simulink model "Predefined_with_GroundTruth_mod1helper"  (R2021b)
settings: Solver=VariableStepAuto  StartTime=0.0  StopTime=inf  RelTol=1e-3
model workspace (MAT data in the model file):
  firstWarning = 1
  originalScenarioChecksum = '114339432DE22364D47BB28FC96DC10C'
undefined symbols (not defined in the file): Acceleration, ActorID, AngularVelocity, curvature, curvature1, curvatureAhd, DefaultGear, DEND_B, DEND_S, DEND_T, direction, driving, EgoRefPose, gradbp, L, LF, LR, matlabshared, MAX_BRAKE, MAX_STEER, MAX_TORQUE, MCAR, MIN_BRAKE, MIN_STEER, MIN_TORQUE, NUMD_B, NUMD_S, NUMD_T, Pitch, Position, psi_o, R, Roll, RRdamp, scenario, SceneInfo, sigbuilder_block, STEER_RATIO, stopSign_ID, Tdead, thetaRefs, TL_ID, TrackWidth, Ts, ts, Vdead, Velocity, VelProfile, X_o, xRef2s, Y_o, Yaw, yRef2s
libraries: drivingscenarioandsensors x8, drivingvehiclecontroller x2, simulink x2, trackingutilitieslib x2, mpcadaslib x1, robotalgslib x1, simulink_extras x1, drivinglib x1, autolibshared x1, vehdynlibviscommon x1, vehdynlibsteering x1
(part 1 of 3)
settings Model: Creator=akshran  LastModifiedBy=almudhaf.3

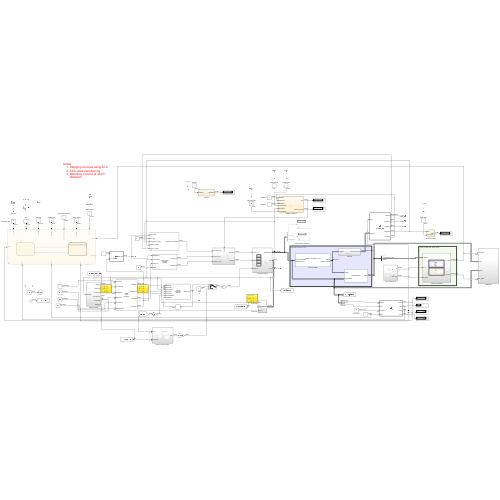
[thumbnail: Simulink's stored preview of the top-level diagram]
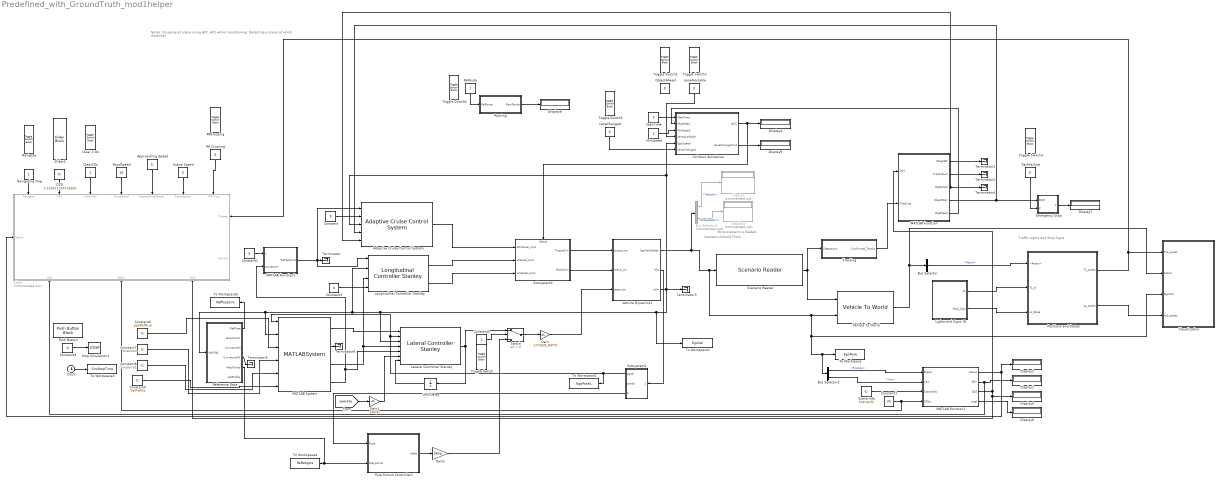
== system Predefined_with_GroundTruth_mod1helper ==
  note: Notes:
      | Stopping at scene using ACC.
      | ACC while transitioning.
      | Detecting a scene at which distance?
  note: Mcity scenario is loaded
  note: Traffic Lights and Stop Signs
  note: Scenario Ground Truth
  Adaptive Cruise Control System : mpcadaslib/Adaptive Cruise Control System  EgoModel=tf(1,[0.5,1,0])  InitialEgoVelocity=0  DefaultSpacing=2  MaxVelocity=50  MinAcceleration=-6  amin_ext=off  MaxAcceleration=6  amax_ext=off  Ts=0.1  PredictionHorizon=30  ControllerBehavior=0.500  suboptimal=off  maxiter=10  datatypeopt=double  optmode=off  trackmode=off
  Approaching Speed : Constant  Value=5
  Bus Selector : BusSelector  OutputSignals=Actors
  Bus Selector2 : BusSelector  OutputSignals=Position,Yaw
  Bus Selector4 : BusSelector  Commented=on  OutputSignals=Velocity,Acceleration
  Chart : Stateflow chart  Commented=on  TreatAsAtomicUnit=on
      settings: PortSchema="{\"entries\":[{\"content\":{\"sides\":[{\"content\":{\"connectorIds\":[\"In8\"]},\"type\":\"ConnectorPlacement.EquallySpacedRectSide\",\"uuid\":\"81aca70f-0947-49fb-b60a-be241e44193b\"},{\"content\":{\"connectorIds\":[\"In1\",\"Out1\"],\"side\":\"RIGHT\"},\"type\":\"ConnectorPlacement.EquallySpacedRectSide\",\"uuid\":\"e7b9645e-3711-4964-ac9b-0199dd335e99\"},{\"content\":{\"connectorIds\":[\"In9\",\"In10\",\"In11\",\"In12\",\"In3\",\"In4\",\"In6\"],\"side\":\"TOP\"},\"type\":\"ConnectorPlacement.EquallySpacedRectSide\",\"uuid\":\"6876f024-944b-4540-9404-d68f37763657\"},{\"content\":{\"connectorIds\":[\"In2\",\"In5\",\"In7\"],\"side\":\"BOTTOM\"},\"type\":\"ConnectorPlacement.EquallySpacedRectSide\",\"uuid\":\"44acab73-cdde-4edf-95df-27422644ccab\"}]},\"type\":\"ConnectorPlacement.EquallySpacedConnector\",\"uuid\":\"d2c31c01-e447-43db-8d2b-8b98a0ca291a\"}],\"packageUris\":[\"http://schema.mathworks.com/mf0/Connector/R2020b\"],\"version\":\"1.0\"}"
  Clear 2 Go : ToggleSwitchBlock
      settings: Values={{'Off', 'On'}, [0 1]}
  Clear2Go : Constant
  Clock : Clock
  Collision Avoidance : Stateflow chart  TreatAsAtomicUnit=on
  Constant : Constant  Value=0
  Constant1 : Constant  Value=25
  Constant2 : Constant  Value=5
  Constant3 : Constant  Value=0
  Constant4 : Constant  Value=0
  Constant5 : Constant
  Constant6 : Constant  Value=EgoRefPose
  Constant7 : Constant  Value=direction
  Constant8 : Constant  Value=curvature1
  Constant9 : Constant  Value=VelProfile
  D2D : Constant  Value=2.529411764705882
  Display : Display  Commented=on
  Display{1..2,4..9} (8 alike) : Display
  Display3 : Display  Commented=on
  Emergency Stop : Stateflow chart  TreatAsAtomicUnit=on
  Gain : Gain  Gain=1/STEER_RATIO
  Gain1 : Gain  Gain=180/pi
  Gain2 : Gain  Gain=180/pi
  LaneAvailable : Constant  Value=0
  LaneChanged : Constant  Value=0
  Lateral Controller Stanley : drivingvehiclecontroller/Lateral Controller Stanley  ModelType=Dynamic bicycle model  PositionGainF=2.5  PositionGainR=2.5  YawRateGain=0.4  DelayGain=0.4  VehicleMass=MCAR  Lf=LF  Lr=LR  TireStiffness=5e3  Wheelbase=3  MaxSteeringAngle=80
      settings: SourceProductBaseCode=DR
  Lights and Signs ID : Subsystem
  Longitudinal Controller Stanley : drivingvehiclecontroller/Longitudinal Controller Stanley  Kp=10  Ki=0.1  SampleTime=0.05  MaxAcceleration=40  MaxDeceleration=40
      settings: SourceProductBaseCode=DR
  MATLAB Function : MATLAB Function  TreatAsAtomicUnit=on
  MATLAB Function1 : MATLAB Function  TreatAsAtomicUnit=on
  MATLAB Function2 : MATLAB Function  TreatAsAtomicUnit=on
  MATLAB System : MATLABSystem  System=HelperPathAnalyzer  Wheelbase=WB  HasResetOutput=off  SimulateUsing=Interpreted execution
      mask Type: HelperPathAnalyzer
      mask Display:
      | disp(['Helper' char(10) 'Path' char(10) 'Analyzer']);
      | port_label('input',1,'CurrPose');
      | port_label('input',2,'CurrVelocity');
      | port_label('input',3,'RefPoses');
      | port_label('input',4,'Directions');
      | port_label('input',5,'Curvatures');
      | port_label('input',6,'RefVelocities');
      | port_label('output',1,'RefPose');
      | port_label('output',2,'RefVelocity');
      | port_label('output',3,'Direction');
      | port_label('output',4,'Curvature');
  MinSpeed : Constant  Value=2
  Navigate : ToggleSwitchBlock
      settings: Values={{'Off', 'On'}, [0 1]}
  Navigating Flag : Constant
  ObjectAhead : Constant  Value=0
  "Positions and States " : Subsystem
  Pure Pursuit Controller1 : Subsystem
  Push Button : PushButtonBlock  OffValue=0.000000
  RR Crossing : Constant  Value=0
  RRCrossing : ToggleSwitchBlock
      settings: Values={{'Off', 'On'}, [0 1]}
  ReRoute : Constant
  Reference Data : Subsystem  VariantControl=Stanley
  RoadSpeed : Constant  Value=15
  Routing : Stateflow chart  TreatAsAtomicUnit=on
  Scenario Reader : drivingscenarioandsensors/Scenario Reader  ScenarioSource=From file  ScenarioFileName=\\coeit.osu.edu\home\a\almudhaf.3\Documents\MATLAB Drive\AutoDrive Challenge II\ad2_y1_simulationpkg_(2)\ad2_y1_simulationpkg\scenarios\scenario_Controllers_test.mat  ScenarioVariableName=scenario  OutputCoordinateSystem=Vehicle coordinates  EgoVehicleSource=Input port  EgoVehicleActorID=1  OrientVehiclesOnRoad=on  OutputEgoVehiclePose=on  OutputEgoVehicleState=off  SampleTime=Ts  LaneBoundaryOutput=None  LaneBoundaryDistance=0:0.5:9.5  LaneBoundaryLocation=Center of lane markings  BusNameSource=Auto  BusName=BusActors  BusNumActorsSource=Scenario  BusNumActors=100  BusName2Source=Auto  BusName2=BusLaneBoundaries  BusNumLaneBoundariesSource=Scenario  BusNumLaneBoundaries=10  BusName3Source=Auto  BusName3=BusEgoActor  BusName4Source=Auto  BusName4=BusEgoState  ShowCoordinateLabels=on  SimulateUsing=Interpreted execution
  Scene Info : Constant  Value=SceneInfo  VectorParams1D=off
  Scene Speed : Constant  Value=5
  Slider1 : SliderBlock  ScaleMax=5
  Stop Simulation1 : Stop
  Subsystem1 : Subsystem
  Subsystem3 : Subsystem
      settings: PortSchema="{\"entries\":[{\"content\":{\"sides\":[{\"content\":{\"connectorIds\":[\"In1\",\"In2\",\"In3\"]},\"type\":\"ConnectorPlacement.EquallySpacedRectSide\",\"uuid\":\"a23b1a10-3bcb-40a0-900c-c9a3f160b173\"},{\"content\":{\"connectorIds\":[\"Out1\",\"Out2\"],\"side\":\"RIGHT\"},\"type\":\"ConnectorPlacement.EquallySpacedRectSide\",\"uuid\":\"88840b66-912f-4184-aeec-297642319416\"},{\"content\":{\"connectorIds\":[\"In4\"],\"side\":\"TOP\"},\"type\":\"ConnectorPlacement.EquallySpacedRectSide\",\"uuid\":\"37a03ca9-b065-473e-b290-3b07703c6005\"}]},\"type\":\"ConnectorPlacement.EquallySpacedConnector\",\"uuid\":\"5bfc7c71-8f7a-4cba-a168-7eeca22a2fcb\"}],\"packageUris\":[\"http://schema.mathworks.com/mf0/Connector/R2020b\"],\"version\":\"1.0\"}"
  Switch : Switch  Criteria=u2 > Threshold
  TechFailure : Constant  Value=0
  Terminator{,1..6} (7 alike) : Terminator
  To Workspace : ToWorkspace  VariableName=EgoPose  SaveFormat=Timeseries  SampleTime=-1
  To Workspace1 : ToWorkspace  VariableName=EgoVel  SampleTime=-1
      settings: Save2DSignal=2-D array (concatenate along first dimension)
  To Workspace2 : ToWorkspace  VariableName=EgoPose1  SampleTime=-1
      settings: Save2DSignal=2-D array (concatenate along first dimension)
  To Workspace3 : ToWorkspace  VariableName=SimStopTime  SampleTime=-1
      settings: Save2DSignal=2-D array (concatenate along first dimension)
  To Workspace4 : ToWorkspace  VariableName=RefWaypts  SampleTime=-1
      settings: Save2DSignal=2-D array (concatenate along first dimension)
  To Workspace5 : ToWorkspace  VariableName=RefPoseSim  SampleTime=-1
      settings: Save2DSignal=2-D array (concatenate along first dimension)
  Toggle Switch{,1..5} (6 alike) : ToggleSwitchBlock
      settings: Values={{'Off', 'On'}, [0 1]}
  Tracking : Subsystem
  Unit Delay : UnitDelay  SampleTime=-1  HasFrameUpgradeWarning=on
  Vehicle Dynamics1 : Subsystem
  Vehicle To World : drivingscenarioandsensors/Vehicle To World  BusNameSource=Auto  BusName=BusVehicleToWorldActors  SimulateUsing=Interpreted execution
      settings: SourceProductBaseCode=DR
  Visualization : Subsystem
  WaitTime : Constant  Value=3
  wires:
  "Positions and States "/1(TL_poses) -> Chart/1(TLstate), Visualization/1(TL1_poses)
  "Positions and States "/2(ss_poses) -> Visualization/4(ss1_poses)
  Lights and Signs ID/2(Stop_Sign) -> "Positions and States "/3(ss_State)
  Vehicle To World/1 -> Visualization/2(Actors), Bus Selector/1
  Vehicle Dynamics1/1(EgoVehStates) -> Bus Selector4/1, Vehicle To World/2, Bus Selector2/1, To Workspace/1, Visualization/3(EgoInfo), Scenario Reader/1
  Bus Selector/1 -> "Positions and States "/1(<Actors>)  "<Actors>"
  Lights and Signs ID/1(TL) -> "Positions and States "/2(TL_id)
  Scenario Reader/1 -> Tracking/1(Detections), Vehicle To World/1
  Bus Selector2/1 -> MATLAB Function1/1(EVpos)  "<Position>"
  Scene Info/1 -> MATLAB Function1/3(SceneInfo)
  Constant1/1 -> MATLAB Function1/4(SDist), Chart/5(SDist)
  MATLAB Function1/1(Scene) -> Display2/1, Chart/8(Scene)
  MATLAB Function1/2(SDir) -> Display1/1, Chart/2(SDir)
  MATLAB Function1/4(angl) -> Display6/1
  Unit Delay/1 -> Lateral Controller Stanley/7
  Lateral Controller Stanley/1 -> Switch/1, Unit Delay/1
  Vehicle Dynamics1/2(Info) -> Subsystem1/1(VehFdbk)
  Constant3/1 -> Longitudinal Controller Stanley/4
  Bus Selector4/1 -> Display/1  "<Velocity>"
  Bus Selector4/2 -> Display3/1  "<Acceleration>"
  Vehicle Dynamics1/3(xdot) -> To Workspace1/1, Longitudinal Controller Stanley/2, MATLAB System/2, Reference Data/1(VelFdbk), Lateral Controller Stanley/3, Terminator3/1, Collision Avoidance/5(EgoSpeed), Adaptive Cruise Control System/3
  Subsystem1/1(pose) -> To Workspace2/1, MATLAB System/1, Lateral Controller Stanley/2
  [yawrate] -> Gain1/1
  Gain1/1 -> Lateral Controller Stanley/6
  Bus Selector2/2 -> MATLAB Function1/2(yaw)  "<Yaw>"
  Navigating Flag/1 -> Chart/9(Navigate)
  Approaching Speed/1 -> Chart/3(ApproachingSpeed)
  Scene Speed/1 -> Chart/4(SceneSpeed)
  Gain/1 -> Vehicle Dynamics1/3(steer_cm)
  RR Crossing/1 -> Chart/6(RRCross)
  D2D/1 -> Chart/10(D2D)
  Clear2Go/1 -> Chart/11(Clear2Go)
  RoadSpeed/1 -> Chart/12(RoadSpeed)
  MATLAB Function1/3(D2S) -> Chart/7(D2S), Display5/1, MATLAB Function/1(D2S)
  Tracking/1(Confirmed_Tracks) -> MATLAB Function/2(Tracking)
  MATLAB Function/1(ObjectID) -> Terminator1/1
  MATLAB Function/2(TracksNum) -> Terminator2/1
  MATLAB Function/3(ObjRelVel) -> Terminator4/1, Adaptive Cruise Control System/5
  TechFailure/1 -> Emergency Stop/2(TechFailure)
  Emergency Stop/1(EStop) -> Display7/1
  Collision Avoidance/1(ACC) -> Subsystem3/4(Select), Display4/1
  MinSpeed/1 -> Collision Avoidance/3(MinSpeed)
  WaitTime/1 -> Collision Avoidance/1(WaitTime)
  LaneAvailable/1 -> Collision Avoidance/4(LaneAvailable)
  ReRoute/1 -> Routing/1(ReRoute)
  Routing/1(NewRoute) -> Display8/1
  Constant/1 -> Adaptive Cruise Control System/2
  LaneChanged/1 -> Collision Avoidance/6(LaneChanged)
  Collision Avoidance/2(LaneChangeCmd) -> Display9/1
  MATLAB Function/5(ObjAhead) -> Collision Avoidance/2(ObjAhead)
  MATLAB Function/4(ObjectDist) -> Emergency Stop/1(D2O), Adaptive Cruise Control System/4
  Adaptive Cruise Control System/1 -> Subsystem3/1(ACCaccel_cmd)
  Longitudinal Controller Stanley/1 -> Subsystem3/2(LCaccel_cmd)
  Longitudinal Controller Stanley/2 -> Subsystem3/3(LCdeccel_cmd)
  Subsystem3/1(TorgueCm) -> Vehicle Dynamics1/1(torque_cm)
  Subsystem3/2(BrakeCm) -> Vehicle Dynamics1/2(brake_cm)
  MATLAB Function2/1(RefVelCmd) -> Adaptive Cruise Control System/1, Longitudinal Controller Stanley/1, Terminator/1
  Clock/1 -> To Workspace3/1
  Reference Data/4(CurvatureO1) -> Terminator5/1
  Constant4/1 -> Stop Simulation1/1
  Constant2/1 -> MATLAB Function2/1(v)
  Pure Pursuit Controller1/1(delta) -> Gain2/1
  Gain2/1 -> Switch/3
  Reference Data/5(WayPoints) -> Pure Pursuit Controller1/2(Waypoints), To Workspace4/1
  Subsystem1/3(PPpose) -> Pure Pursuit Controller1/1(Pose)
  Constant5/1 -> Switch/2
  Switch/1 -> Gain/1
  MATLAB System/4 -> MATLAB Function2/2(curvature), Lateral Controller Stanley/5
  MATLAB System/3 -> Longitudinal Controller Stanley/3, Lateral Controller Stanley/4
  MATLAB System/1 -> Lateral Controller Stanley/1
  MATLAB System/2 -> Terminator6/1
  Constant6/1 -> MATLAB System/3
  Constant7/1 -> MATLAB System/4
  Constant8/1 -> MATLAB System/5
  Constant9/1 -> MATLAB System/6
  Reference Data/1(RefPose) -> To Workspace5/1

== system Predefined_with_GroundTruth_mod1helper/Lights and Signs ID ==
  Constant : Constant  Value=TL_ID
  Constant1 : Constant  Value=stopSign_ID
  TL : Outport
  Stop_Sign : Outport  Port=2
  wires:
  Constant/1 -> TL/1
  Constant1/1 -> Stop_Sign/1

== system Predefined_with_GroundTruth_mod1helper/Positions and States  ==
  note: Stop Sign positon
  note: Traffic Light Position and State
  <Actors> : Inport
  TL_id : Inport  Port=2
  ss_State : Inport  Port=3
  MATLAB Function1 : MATLAB Function  TreatAsAtomicUnit=on
  MATLAB Function2 : MATLAB Function  TreatAsAtomicUnit=on
  Traffic Light Sensor : Subsystem  mask{TrafficLightSensorModeSelection=Cycle}
      mask prompts: TrafficLightSensorModeSelection "Traffic Light Sensor Mode:"
      mask TypeOptions TrafficLightSensorModeSelection: Steady Green | Steady Red | Cycle
      mask DialogControl DescTextVar Prompt: Simulate a traffic light sensor.
  TL_poses : Outport
  ss_poses : Outport  Port=2
  wires:
  <Actors>/1 -> MATLAB Function2/1(Actors), MATLAB Function1/1(Actors)
  ss_State/1 -> MATLAB Function2/2(ss_State)
  TL_id/1 -> Traffic Light Sensor/1(TL_id)
  Traffic Light Sensor/1(TL_State) -> MATLAB Function1/2(TL_State)  "TL_State"
  MATLAB Function2/1(ss_poses) -> ss_poses/1
  MATLAB Function1/1(TL_poses) -> TL_poses/1

== system Predefined_with_GroundTruth_mod1helper/Pure Pursuit Controller1 ==
  note: The subsystem implements a Pure Pursuit controller. The "Pure Pursuit" block calculates the target direction and the "Wheel Steering Angle Formulation" block calculates the wheel steering angle.
  Pose : Inport
  Waypoints : Inport  Port=2
  Pure Pursuit : robotalgslib/Pure Pursuit  DesiredLinearVelocity=1  MaxAngularVelocity=1.0  LookaheadDistance=10  TargetDirPort=on  SimulateUsing=Code generation
  Terminator6 : Terminator
  Terminator7 : Terminator
  Wheel Steering Angle Formulation : Subsystem  mask{L=L, ld=10}
      mask prompts: L "Bicycle length"; ld "Lookahead distance"
      mask TypeOptions L: Bicycle length/Value
      mask TypeOptions ld: Lookahead distance/Value
      mask Display:
      | image("GeometryMask.png")
      | port_label('input', 1, 'alpha')
      | port_label('output', 1, 'delta')
  delta : Outport
  wires:
  Wheel Steering Angle Formulation/1(Al) -> delta/1
  Pure Pursuit/3 -> Wheel Steering Angle Formulation/1(alpha)
  Pure Pursuit/2 -> Terminator7/1
  Pose/1 -> Pure Pursuit/1
  Pure Pursuit/1 -> Terminator6/1
  Waypoints/1 -> Pure Pursuit/2

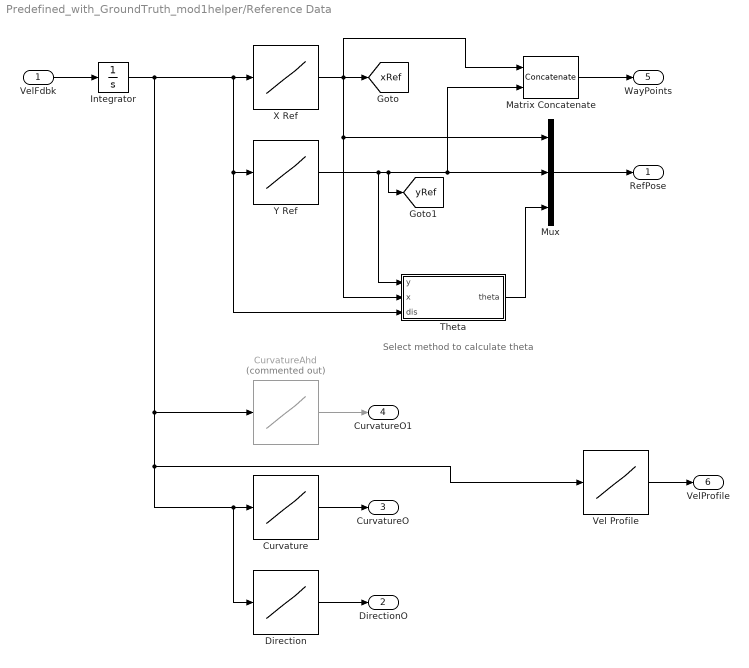
== system Predefined_with_GroundTruth_mod1helper/Reference Data ==
  note: Select method to calculate theta
  VelFdbk : Inport
  Curvature : Lookup_n-D  NumberOfTableDimensions=1  BreakpointsForDimension1=gradbp  Table=curvature  InternalRulePriority=Speed  RndMeth=Simplest  InputSameDT=on
  CurvatureAhd : Lookup_n-D  Commented=on  NumberOfTableDimensions=1  BreakpointsForDimension1=gradbp  Table=curvatureAhd  InternalRulePriority=Speed  RndMeth=Simplest  InputSameDT=on
  Direction : Lookup_n-D  NumberOfTableDimensions=1  BreakpointsForDimension1=gradbp  Table=direction  InternalRulePriority=Speed  RndMeth=Simplest  InputSameDT=on
  Integrator : Integrator
  Matrix Concatenate : Concatenate  Mode=Multidimensional array  ConcatenateDimension=2
  Mux : Mux  Inputs=3
  Theta : Subsystem  Variant=on  VariantControlMode=label  LabelModeActiveChoice=thetaLookUpTable
  Vel Profile : Lookup_n-D  NumberOfTableDimensions=1  BreakpointsForDimension1=gradbp  Table=VelProfile  InternalRulePriority=Speed  RndMeth=Simplest  InputSameDT=on
  X Ref : Lookup_n-D  NumberOfTableDimensions=1  BreakpointsForDimension1=gradbp  Table=xRef2s  InternalRulePriority=Speed  RndMeth=Simplest  InputSameDT=on
  Y Ref : Lookup_n-D  NumberOfTableDimensions=1  BreakpointsForDimension1=gradbp  Table=yRef2s  InternalRulePriority=Speed  RndMeth=Simplest  InputSameDT=on
  RefPose : Outport
  DirectionO : Outport  Port=2
  CurvatureO : Outport  Port=3
  CurvatureO1 : Outport  Port=4
  WayPoints : Outport  Port=5
  VelProfile : Outport  Port=6
  tag scope: xRef=global, yRef=global
  wires:
  Direction/1 -> DirectionO/1
  Curvature/1 -> CurvatureO/1
  Mux/1 -> RefPose/1
  Integrator/1 -> Curvature/1, Direction/1, Vel Profile/1, CurvatureAhd/1, Theta/3(dis), Y Ref/1, X Ref/1
  VelFdbk/1 -> Integrator/1
  Theta/1(theta) -> Mux/3
  CurvatureAhd/1 -> CurvatureO1/1
  Matrix Concatenate/1 -> WayPoints/1
  X Ref/1 -> Theta/2(x), Mux/1, Matrix Concatenate/1, [xRef]
  Y Ref/1 -> Theta/1(y), Matrix Concatenate/2, Mux/2, [yRef]
  Vel Profile/1 -> VelProfile/1

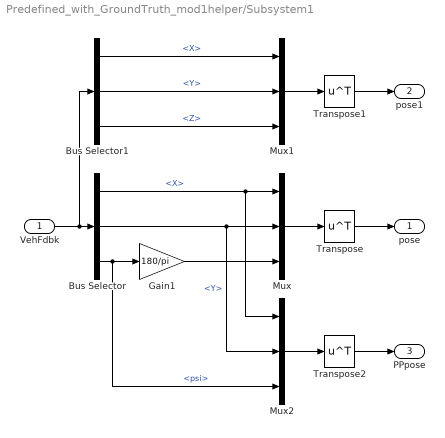
== system Predefined_with_GroundTruth_mod1helper/Subsystem1 ==
  VehFdbk : Inport
  Bus Selector : BusSelector  OutputSignals=InertFrm.Cg.Disp.X,InertFrm.Cg.Disp.Y,InertFrm.Cg.Ang.psi
  Bus Selector1 : BusSelector  OutputSignals=InertFrm.Cg.Disp.X,InertFrm.Cg.Disp.Y,InertFrm.Cg.Disp.Z
  Gain1 : Gain  Gain=180/pi
  Mux : Mux  Inputs=3
  Mux1 : Mux  Inputs=3
  Mux2 : Mux  Inputs=3
  Transpose : Math  Operator=transpose  SignedPower=on  SaturateOnIntegerOverflow=on
  Transpose1 : Math  Operator=transpose  SignedPower=on  SaturateOnIntegerOverflow=on
  Transpose2 : Math  Operator=transpose  SignedPower=on  SaturateOnIntegerOverflow=on
  pose : Outport
  pose1 : Outport  Port=2
  PPpose : Outport  Port=3
  wires:
  Mux/1 -> Transpose/1
  VehFdbk/1 -> Bus Selector1/1, Bus Selector/1
  Gain1/1 -> Mux/3
  Transpose/1 -> pose/1
  Bus Selector/3 -> Mux2/3, Gain1/1  "<psi>"
  Bus Selector1/1 -> Mux1/1  "<X>"
  Bus Selector1/2 -> Mux1/2  "<Y>"
  Bus Selector1/3 -> Mux1/3  "<Z>"
  Mux1/1 -> Transpose1/1
  Transpose1/1 -> pose1/1
  Mux2/1 -> Transpose2/1
  Transpose2/1 -> PPpose/1
  Bus Selector/2 -> Mux/2, Mux2/2  "<Y>"
  Bus Selector/1 -> Mux/1, Mux2/1  "<X>"

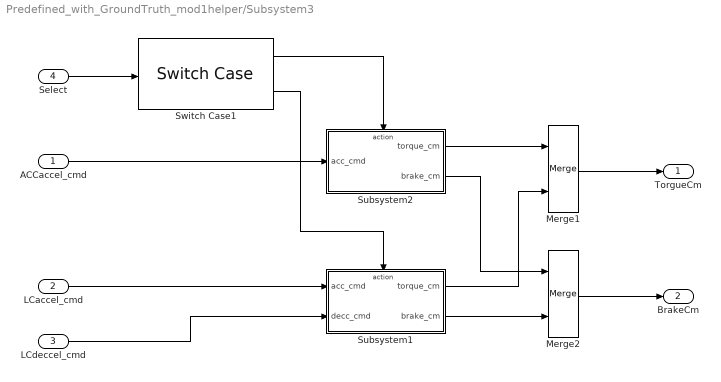
== system Predefined_with_GroundTruth_mod1helper/Subsystem3 ==
  ACCaccel_cmd : Inport
  LCaccel_cmd : Inport  Port=2
  LCdeccel_cmd : Inport  Port=3
  Select : Inport  Port=4
  Merge1 : Merge
  Merge2 : Merge
  Subsystem1 : Subsystem
  Subsystem2 : Subsystem
  Switch Case1 : SwitchCase  CaseConditions={1, 0}  ShowDefaultCase=off
  TorgueCm : Outport
  BrakeCm : Outport  Port=2
  wires:
  LCdeccel_cmd/1 -> Subsystem1/2(decc_cmd)
  Subsystem1/2(brake_cm) -> Merge2/2
  Subsystem1/1(torque_cm) -> Merge1/2
  Subsystem2/2(brake_cm) -> Merge2/1
  Switch Case1/1 -> Subsystem2/Action
  Switch Case1/2 -> Subsystem1/Action
  Subsystem2/1(torque_cm) -> Merge1/1
  LCaccel_cmd/1 -> Subsystem1/1(acc_cmd)
  Merge2/1 -> BrakeCm/1
  ACCaccel_cmd/1 -> Subsystem2/1(acc_cmd)
  Merge1/1 -> TorgueCm/1
  Select/1 -> Switch Case1/1

== system Predefined_with_GroundTruth_mod1helper/Tracking ==
  Detections : Inport
  Camera : drivingscenarioandsensors/Vision Detection Generator  SensorIndex=1  DetectorOutput=Objects only  UpdateInterval=0.01  LaneUpdateInterval=0.1  SensorLocation=[1.9 0]  Height=1.1  Yaw=0  Pitch=1  Roll=0  BusNameSource=Auto  BusName=BusObjectDetections  BusName2Source=Auto  BusName2=BusLaneDetections  MaxNumDetectionsSource=Property  MaxNumDetections=10  MaxNumLanesSource=Property  MaxNumLanes=30  DetectionCoordinates=Ego Cartesian  SimulateUsing=Interpreted execution  MaxRange=150  BoundingBoxAccuracy=5  ProcessNoiseIntensity=5  MaxSpeed=100  MaxAllowedOcclusion=0.5  MinObjectImageSize=[1 1]  DetectionProbability=0.9  FalsePositivesPerImage=0.1  MinLaneImageSize=[20 3]  LaneBoundaryAccuracy=3  HasNoise=on  InitialSeedSource=Repeatable  InitialSeed=0  UsedSeed=0  ActorProfilesSource=From Scenario Reader block  ActorProfilesParameters=driving.internal.ActorProfilesParameters  ActorProfilesExpression=[struct('ActorID',1,'ClassID',1,'Length',4.7,'Width',1.8,'Height',1.4,'OriginOffset',[-1.35 0 0],'MeshVertices',[3.7 0.9 0.857439446366782;3.7 -0.9 0.857439446366782;3.7 -0.9 0.314878892733564;3.7 0.9 0.314878892733564;3.7 0.9 0.857439446366782;2.525 0.9 0.993079584775086;2.525 -0.9 0.993079584775086;3.7 -0.9 0.857439446366782;1.82 0.72 1.4;0.41 0.72 1.4;0.41 -0.72 1.4;1.82 -0.72 1.4;-0.295 0.9 0.993079584775086;-1 0.9 0.857439446366782;-1 -0.9 0.857439446366782;-0.295 -0.9 0.993079584775086;3.7 0.9 0.857439446366782;3.7 0.9 0.314878892733564;2.525 0.9 0.314878892733564;2.525 0.9 0.993079584775086;2.525 0.9 0.993079584775086;2.525 0.9 0.314878892733564;-0.295 0.9 0.314878892733564;-0.295 0.9 0.993079584775086;-0.295 0.9 0.993079584775086;-0.295 0.9 0.314878892733564;-1 0.9 0.355570934256055;-1 0.9 0.857439446366782;2.525 0.9 0.993079584775086;-0.295 0.9 0.993079584775086;0.41 0.72 1.4;1.82 0.72 1.4;3.7 -0.9 0.857439446366782;3.7 -0.9 0.314878892733564;2.525 -0.9 0.314878892733564;2.525 -0.9 0.993079584775086;2.525 -0.9 0.993079584775086;2.525 -0.9 0.314878892733564;-0.295 -0.9 0.314878892733564;-0.295 -0.9 0.993079584775086;-0.295 -0.9 0.993079584775086;-0.295 -0.9 0.314878892733564;-1 -0.9 0.355570934256055;-1 -0.9 0.857439446366782;2.525 -0.9 0.993079584775086;-0.295 -0.9 0.993079584775086;0.41 -0.72 1.4;1.82 -0.72 1.4;-0.295 0.9 0.993079584775086;-0.295 -0.9 0.993079584775086;0.41 -0.72 1.4;0.41 0.72 1.4;2.525 -0.9 0.993079584775086;1.82 -0.72 1.4;1.82 0.72 1.4;2.525 0.9 0.993079584775086;-1 0.9 0.857439446366782;-1 0.9 0.355570934256055;-1 -0.9 0.355570934256055;-1 -0.9 0.857439446366782;3.7 0.9 0.314878892733564;3.7 -0.9 0.314878892733564;-0.295 -0.9 0.314878892733564;-0.295 0.9 0.314878892733564;-0.295 0.9 0.314878892733564;-1 0.9 0.355570934256055;-1 -0.9 0.355570934256055;-0.295 -0.9 0.314878892733564;0 -0.63 0;0 -0.87 0;0.191030206995054 -0.63 0.0601365173421445;0.191030206995054 -0.87 0.0601365173421445;0.309093367795925 -0.63 0.217575963708927;0.309093367795925 -0.87 0.217575963708927;0.309093367795925 -0.63 0.412181821758201;0.309093367795925 -0.87 0.412181821758201;0.191030206995054 -0.63 0.569621268124983;0.191030206995054 -0.87 0.569621268124983;0 -0.63 0.629757785467128;0 -0.87 0.629757785467128;-0.191030206995054 -0.63 0.569621268124983;-0.191030206995054 -0.87 0.569621268124983;-0.309093367795925 -0.63 0.412181821758201;-0.309093367795925 -0.87 0.412181821758201;-0.309093367795925 -0.63 0.217575963708927;-0.309093367795925 -0.87 0.217575963708927;-0.191030206995054 -0.63 0.0601365173421445;-0.191030206995054 -0.87 0.0601365173421445;0 -0.63 0;0 -0.87 0;0 -0.63 0;0.191030206995054 -0.63 0.0601365173421445;0.309093367795925 -0.63 0.217575963708927;0.309093367795925 -0.63 0.412181821758201;0.191030206995054 -0.63 0.569621268124983;0 -0.63 0.629757785467128;-0.191030206995054 -0.63 0.569621268124983;-0.309093367795925 -0.63 0.412181821758201;-0.309093367795925 -0.63 0.217575963708927;-0.191030206995054 -0.63 0.0601365173421445;0 -0.87 0;0.191030206995054 -0.87 0.0601365173421445;0.309093367795925 -0.87 0.217575963708927;0.309093367795925 -0.87 0.412181821758201;0.191030206995054 -0.87 0.569621268124983;0 -0.87 0.629757785467128;-0.191030206995054 -0.87 0.569621268124983;-0.309093367795925 -0.87 0.412181821758201;-0.309093367795925 -0.87 0.217575963708927;-0.191030206995054 -0.87 0.0601365173421445;0 0.87 0;0 0.63 0;0.191030206995054 0.87 0.0601365173421445;0.191030206995054 0.63 0.0601365173421445;0.309093367795925 0.87 0.217575963708927;0.309093367795925 0.63 0.217575963708927;0.309093367795925 0.87 0.412181821758201;0.309093367795925 0.63 0.412181821758201;0.191030206995054 0.87 0.569621268124983;0.191030206995054 0.63 0.569621268124983;0 0.87 0.629757785467128;0 0.63 0.629757785467128;-0.191030206995054 0.87 0.569621268124983;-0.191030206995054 0.63 0.569621268124983;-0.309093367795925 0.87 0.412181821758201;-0.309093367795925 0.63 0.412181821758201;-0.309093367795925 0.87 0.217575963708927;-0.309093367795925 0.63 0.217575963708927;-0.191030206995054 0.87 0.0601365173421445;-0.191030206995054 0.63 0.0601365173421445;0 ...(+3718 chars)],'MeshFaces',[1 2 3;3 4 1;5 6 7;7 8 5;9 10 11;11 12 9;13 14 15;15 16 13;17 18 19;19 20 17;21 22 23;23 24 21;25 26 27;27 28 25;29 30 31;31 32 29;33 34 35;35 36 33;37 38 39;39 40 37;41 42 43;43 44 41;45 46 47;47 48 45;49 50 51;51 52 49;53 54 55;55 56 53;57 58 59;59 60 57;61 62 63;63 64 61;65 66 67;67 68 65;69 71 72;72 70 69;71 73 74;74 72 71;73 75 76;76 74 73;75 77 78;78 76 75;77 79 80;80 78 77;79 81 82;82 80 79;81 83 84;84 82 81;83 85 86;86 84 83;85 87 88;88 86 85;87 89 90;90 88 87;91 92 93;91 93 94;91 94 95;91 95 96;91 96 97;91 97 98;91 98 99;91 99 100;101 102 103;101 103 104;101 104 105;101 105 106;101 106 107;101 107 108;101 108 109;101 109 110;111 113 114;114 112 111;113 115 116;116 114 113;115 117 118;118 116 115;117 119 120;120 118 117;119 121 122;122 120 119;121 123 124;124 122 121;123 125 126;126 124 123;125 127 128;128 126 125;127 129 130;130 128 127;129 131 132;132 130 129;133 134 135;133 135 136;133 136 137;133 137 138;133 138 139;133 139 140;133 140 141;133 141 142;143 144 145;143 145 146;143 146 147;143 147 148;143 148 149;143 149 150;143 150 151;143 151 152;153 155 156;156 154 153;155 157 158;158 156 155;157 159 160;160 158 157;159 161 162;162 160 159;161 163 164;164 162 161;163 165 166;166 164 163;165 167 168;168 166 165;167 169 170;170 168 167;169 171 172;172 170 169;171 173 174;174 172 171;175 176 177;175 177 178;175 178 179;175 179 180;175 180 181;175 181 182;175 182 183;175 183 184;185 186 187;185 187 188;185 188 189;185 189 190;185 190 191;185 191 192;185 192 193;185 193 194;195 197 198;198 196 195;197 199 200;200 198 197;199 201 202;202 200 199;201 203 204;204 202 201;203 205 206;206 204 203;205 207 208;208 206 205;207 209 210;210 208 207;209 211 212;212 210 209;211 213 214;214 212 211;213 215 216;216 214 213;217 218 219;217 219 220;217 220 221;217 221 222;217 222 223;217 223 224;217 224 225;217 225 226;227 228 229;227 229 230;227 230 231;227 231 232;227 232 233;227 233 234;227 234 235;227 235 236],'RCSPattern',[10 10;10 10],'RCSAzimuthAngles',[-180 180],'RCSElevationAngles',[-90 90]); struct('ActorID',2,'ClassID',7,'Length',0.7,'Width',0.2,'Height',0.1,'OriginOffset',[0 0 0],'MeshVertices',[0.35 -0.1 0.1;0.35 0.1 0.1;-0.35 0.1 0.1;-0.35 -0.1 0.1;0.35 -0.1 0;0.35 0.1 0;-0.35 0.1 0;-0.35 -0.1 0],'MeshFaces',[6 2 1;1 5 6;8 4 3;3 7 8;6 7 3;3 2 6;5 1 4;4 8 5;4 1 2;2 3 4;7 6 5;5 8 7],'RCSPattern',[10 10;10 10],'RCSAzimuthAngles',[-180 180],'RCSElevationAngles',[-90 90])]  Intrinsics=driving.internal.cameraIntrinsics('FocalLength',[400 800],'PrincipalPoint',[320 240],'ImageSize',[480 640],'RadialDistortion',[0 0],'TangentialDistortion',[0 0],'Skew',0)
  Detection Concatenation : trackingutilitieslib/Detection Concatenation  NumInputs=2  BusNameSource=Property  BusName=Detections  SimulateUsing=Interpreted execution
      settings: SourceProductBaseCode=AE,DR,TF,RA,UV,VE
  Multi-Object Tracker : drivinglib/Multi-Object Tracker  TrackerIndex=uint32( 0 )  FilterInitializationFcn=helperInitSimulinkDemoFilter  AssignmentThreshold=50  ConfirmationThreshold=[ 2, 3 ]  DeletionThreshold=[ 5, 5 ]  MaxNumTracks=20  MaxNumSensors=20  OOSMHandling=Neglect  StateParametersSimulink=struct  HasStateParametersInput=off  TimeInputSource=Auto  HasCostMatrixInput=off  HasDetectableTrackIDsInput=off  BusNameSource=Auto  BusName=BusMultiObjectTracker  TentativeTracksOutputPort=off  AllTracksOutputPort=off  SimulateUsing=Interpreted execution
      settings: SourceProductBaseCode=DR
  Radar Detection Generator : drivingscenarioandsensors/Radar Detection Generator  SensorIndex=2  UpdateInterval=0.01  SensorLocation=[ 1.5, 0 ]  Height=0.2  Yaw=0  Pitch=0  Roll=0  BusNameSource=Auto  BusName=BusRadarDetectionGenerator  MaxNumDetectionsSource=Property  MaxNumDetections=50  DetectionCoordinates=Ego Cartesian  SimulateUsing=Interpreted execution  AzimuthResolution=4  ElevationResolution=10  RangeResolution=2.5  RangeRateResolution=0.5  AzimuthBiasFraction=0.1  ElevationBiasFraction=0.1  RangeBiasFraction=0.05  RangeRateBiasFraction=0.05  FieldOfView=[ 60, 5 ]  MaxRange=150  RangeRateLimits=[ -100, 100 ]  DetectionProbability=0.9  FalseAlarmRate=1e-6  ReferenceRange=100  ReferenceRCS=0  HasElevation=off  HasRangeRate=on  HasNoise=on  HasFalseAlarms=on  HasOcclusion=on  InitialSeedSource=Repeatable  InitialSeed=0  UsedSeed=matlabshared.tracking.internal.SimulinkUtilities.seedManager(gcb)  ActorProfilesSource=Parameters  ActorProfilesParameters=driving.internal.ActorProfilesRadarParameters  ActorProfilesExpression=struct( 'ClassID', 0, 'Length', 4.7, 'Width', 1.8, 'Height', 1.4, 'OriginOffset', [ -1.35, 0, 0 ], 'RCSPattern', [ 10, 10; 10, 10 ], 'RCSAzimuthAngles', [ -180, 180 ], 'RCSElevationAngles', [ -90, 90 ] )
      settings: SourceProductBaseCode=DR
  Subsystem1 : Subsystem  Commented=on
  Confirmed_Tracks : Outport
  wires:
  Camera/1 -> Detection Concatenation/1  "Camera Detections"
  Radar Detection Generator/1 -> Detection Concatenation/2  "Lidar Detections"
  Detections/1 -> Radar Detection Generator/1, Camera/1
  Detection Concatenation/1 -> Multi-Object Tracker/1
  Multi-Object Tracker/1 -> Confirmed_Tracks/1

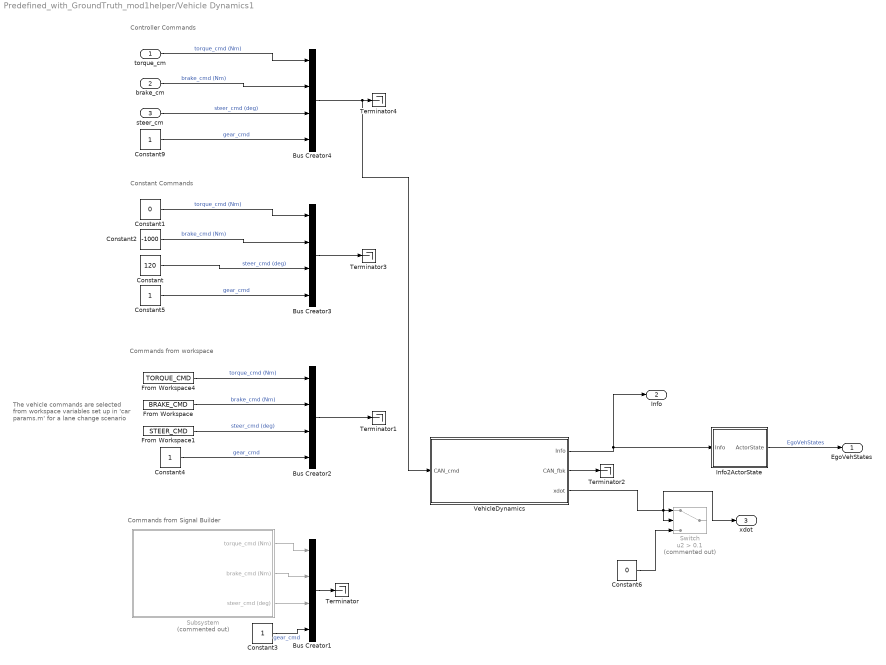
== system Predefined_with_GroundTruth_mod1helper/Vehicle Dynamics1 ==
  note: Constant Commands
  note: Commands from workspace
  note: Commands from Signal Builder
  note: The vehicle commands are selected from workspace variables set up in 'car params.m' for a lane change scenario
  note: Controller Commands
  torque_cm : Inport
  brake_cm : Inport  Port=2
  steer_cm : Inport  Port=3
  Bus Creator{1..4} (4 alike) : BusCreator  Inputs=4
  Constant : Constant  Value=120
  Constant1 : Constant  Value=0
  Constant2 : Constant  Value=-1000
  Constant{3..5,9} (4 alike) : Constant
  Constant6 : Constant  Value=0
  From Workspace : FromWorkspace  VariableName=BRAKE_CMD  SampleTime=ts
  From Workspace1 : FromWorkspace  VariableName=STEER_CMD  SampleTime=ts
  From Workspace4 : FromWorkspace  VariableName=TORQUE_CMD  SampleTime=ts
  Info2ActorState : Subsystem
  Subsystem : Subsystem  Commented=on
  Switch : Switch  Commented=on  Criteria=u2 > Threshold  Threshold=0.1
  Terminator{,1..4} (5 alike) : Terminator
  VehicleDynamics : Subsystem  mask{InitPosition=scenario.Actors(1).Position-0.5*scenario.Actors(1).Wheelbase*[cosd(scenario.Actors(1).Yaw) sind(scenario.Actors(1).Yaw) 0], InitSpeed=norm(scenario.Actors(1).Velocity)*0, InitYaw=(scenario.Actors(1).Yaw/scenario.Actors(1).Yaw)*psi_o}
      mask prompts: InitPosition "Initial Position (m)"; InitSpeed "Initial Speed (m/s)"; InitYaw "Init Yaw (rad)"
  EgoVehStates : Outport
  Info : Outport  Port=2
  xdot : Outport  Port=3
  wires:
  Bus Creator2/1 -> Terminator1/1
  VehicleDynamics/2(CAN_fbk) -> Terminator2/1
  VehicleDynamics/1(Info) -> Info/1, Info2ActorState/1(Info)
  Constant/1 -> Bus Creator3/3  "steer_cmd (deg)"
  Info2ActorState/1(ActorState) -> EgoVehStates/1  "EgoVehStates"
  Constant1/1 -> Bus Creator3/1  "torque_cmd (Nm)"
  Constant2/1 -> Bus Creator3/2  "brake_cmd (Nm)"
  VehicleDynamics/3(xdot) -> Switch/2, Switch/1, xdot/1
  Subsystem/1(torque_cmd (Nm)) -> Bus Creator1/1
  Subsystem/2(brake_cmd (Nm)) -> Bus Creator1/2
  Subsystem/3(steer_cmd (deg)) -> Bus Creator1/3
  Constant3/1 -> Bus Creator1/4  "gear_cmd"
  Constant4/1 -> Bus Creator2/4  "gear_cmd"
  From Workspace/1 -> Bus Creator2/2  "brake_cmd (Nm)"
  From Workspace1/1 -> Bus Creator2/3  "steer_cmd (deg)"
  From Workspace4/1 -> Bus Creator2/1  "torque_cmd (Nm)"
  Constant5/1 -> Bus Creator3/4  "gear_cmd"
  Bus Creator1/1 -> Terminator/1
  brake_cm/1 -> Bus Creator4/2  "brake_cmd (Nm)"
  Constant9/1 -> Bus Creator4/4  "gear_cmd"
  torque_cm/1 -> Bus Creator4/1  "torque_cmd (Nm)"
  steer_cm/1 -> Bus Creator4/3  "steer_cmd (deg)"
  Bus Creator3/1 -> Terminator3/1
  Bus Creator4/1 -> VehicleDynamics/1(CAN_cmd), Terminator4/1
  Constant6/1 -> Switch/3

== system Predefined_with_GroundTruth_mod1helper/Visualization ==
  note: Visualization
  TL1_poses : Inport
  Actors : Inport  Port=2
  EgoInfo : Inport  Port=3
  ss1_poses : Inport  Port=4
  Visualization : MATLABSystem  System=TL_vis
      mask Type: TL_vis
      mask Display:
      | disp('TL_vis');
      | port_label('input',1,'TL');
      | port_label('input',2,'TargetPoses');
      | port_label('input',3,'EgoInfo');
      | port_label('input',4,'SS');
  wires:
  EgoInfo/1 -> Visualization/3
  Actors/1 -> Visualization/2  "target_vehicle_poses"
  TL1_poses/1 -> Visualization/1
  ss1_poses/1 -> Visualization/4

== system Predefined_with_GroundTruth_mod1helper/Positions and States /Traffic Light Sensor ==
  note: Traffic Light Sensor
  TL_id : Inport
  Bus Creator : BusCreator  Inputs=2
  LightConfiguration : Constant  Value=TrafficLightSensorModeSelection
  Traffic Light Switching Logic : Stateflow chart  TreatAsAtomicUnit=on
  TL_State : Outport
  wires:
  LightConfiguration/1 -> Traffic Light Switching Logic/1(LightConfig)
  TL_id/1 -> Traffic Light Switching Logic/2(TL_id)
  Bus Creator/1 -> TL_State/1
  Traffic Light Switching Logic/2(trafficLight) -> Bus Creator/1
  Traffic Light Switching Logic/1(TL_ID) -> Bus Creator/2

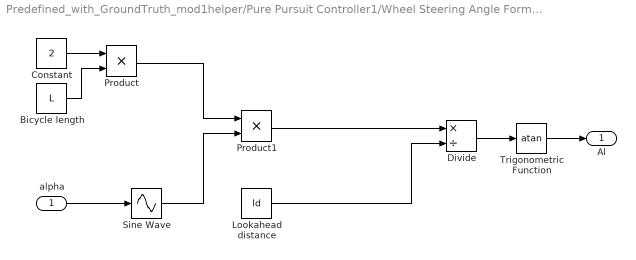
== system Predefined_with_GroundTruth_mod1helper/Pure Pursuit Controller1/Wheel Steering Angle Formulation ==
  alpha : Inport
  Bicycle length : Constant  Value=L
  Constant : Constant  Value=2
  Divide : Product  Inputs=*/
  Lookahead distance : Constant  Value=ld
  Product : Product
  Product1 : Product
  Sine Wave : Sin  TimeSource=Use external signal  SampleTime=0
  Trigonometric Function : Trigonometry  Operator=atan
  Al : Outport
  wires:
  Sine Wave/1 -> Product1/2
  Bicycle length/1 -> Product/2
  Constant/1 -> Product/1
  Product1/1 -> Divide/1
  Product/1 -> Product1/1
  Divide/1 -> Trigonometric Function/1
  Trigonometric Function/1 -> Al/1
  alpha/1 -> Sine Wave/1
  Lookahead distance/1 -> Divide/2

== system Predefined_with_GroundTruth_mod1helper/Reference Data/Theta ==
  note: 1) Add Subsystem or Model blocks as valid variant choices.
      | 2) You cannot connect blocks at this level. At simulation, connectivity is automatically
      | determined, based on the active variant and port name matching.
  y : Inport
  x : Inport  Port=2
  dis : Inport  Port=3
  thetaBlocks : Subsystem  VariantControl=thetaSimulinkBlock
  thetaLt : Subsystem  VariantControl=thetaLookUpTable
  theta : Outport

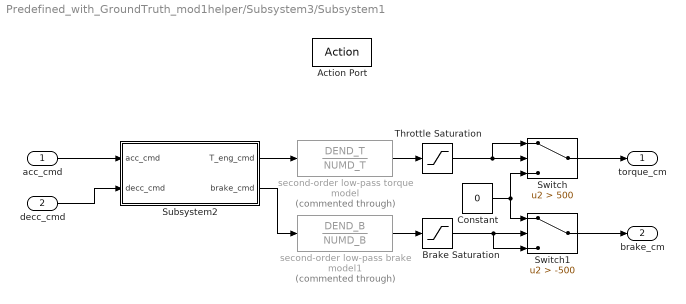
== system Predefined_with_GroundTruth_mod1helper/Subsystem3/Subsystem1 ==
  acc_cmd : Inport
  decc_cmd : Inport  Port=2
  Action Port : ActionPort  ActionPortLabel=case [ 0 ]:
  Brake Saturation : Saturate  UpperLimit=MAX_BRAKE  LowerLimit=MIN_BRAKE
  Constant : Constant  Value=0
  Subsystem2 : Subsystem
  Switch : Switch  Criteria=u2 > Threshold  Threshold=500
  Switch1 : Switch  Criteria=u2 > Threshold  Threshold=-500
  Throttle Saturation : Saturate  UpperLimit=MAX_TORQUE  LowerLimit=MIN_TORQUE
  second-order low-pass brake model1 : DiscreteTransferFcn  Commented=through  Numerator=DEND_B  Denominator=NUMD_B  SampleTime=ts
  second-order low-pass torque model : DiscreteTransferFcn  Commented=through  Numerator=DEND_T  Denominator=NUMD_T  SampleTime=ts
  torque_cm : Outport
  brake_cm : Outport  Port=2
  wires:
  Subsystem2/1(T_eng_cmd) -> second-order low-pass torque model/1
  acc_cmd/1 -> Subsystem2/1(acc_cmd)
  second-order low-pass brake model1/1 -> Brake Saturation/1
  Subsystem2/2(brake_cmd) -> second-order low-pass brake model1/1
  decc_cmd/1 -> Subsystem2/2(decc_cmd)
  second-order low-pass torque model/1 -> Throttle Saturation/1
  Throttle Saturation/1 -> Switch/2, Switch/1
  Switch/1 -> torque_cm/1
  Brake Saturation/1 -> Switch1/2, Switch1/3
  Switch1/1 -> brake_cm/1
  Constant/1 -> Switch/3, Switch1/1

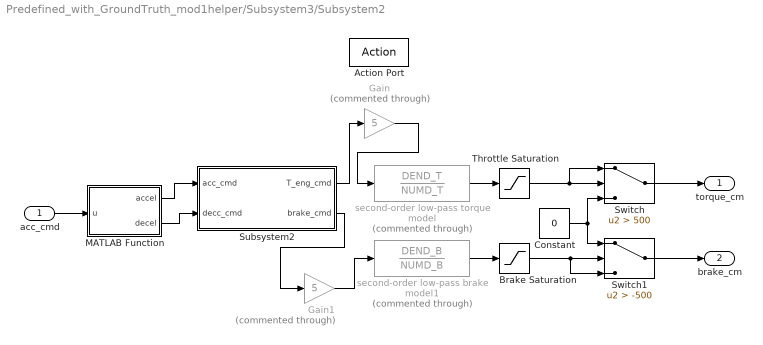
== system Predefined_with_GroundTruth_mod1helper/Subsystem3/Subsystem2 ==
  acc_cmd : Inport
  Action Port : ActionPort  ActionPortLabel=case [ 1 ]:
  Brake Saturation : Saturate  UpperLimit=MAX_BRAKE  LowerLimit=MIN_BRAKE
  Constant : Constant  Value=0
  Gain : Gain  Commented=through  Gain=5
  Gain1 : Gain  Commented=through  Gain=5
  MATLAB Function : MATLAB Function  TreatAsAtomicUnit=on
  Subsystem2 : Subsystem
  Switch : Switch  Criteria=u2 > Threshold  Threshold=500
  Switch1 : Switch  Criteria=u2 > Threshold  Threshold=-500
  Throttle Saturation : Saturate  UpperLimit=MAX_TORQUE  LowerLimit=MIN_TORQUE
  second-order low-pass brake model1 : DiscreteTransferFcn  Commented=through  Numerator=DEND_B  Denominator=NUMD_B  SampleTime=ts
  second-order low-pass torque model : DiscreteTransferFcn  Commented=through  Numerator=DEND_T  Denominator=NUMD_T  SampleTime=ts
  torque_cm : Outport
  brake_cm : Outport  Port=2
  wires:
  second-order low-pass brake model1/1 -> Brake Saturation/1
  second-order low-pass torque model/1 -> Throttle Saturation/1
  Throttle Saturation/1 -> Switch/2, Switch/1
  Switch/1 -> torque_cm/1
  Brake Saturation/1 -> Switch1/2, Switch1/3
  Switch1/1 -> brake_cm/1
  Constant/1 -> Switch/3, Switch1/1
  acc_cmd/1 -> MATLAB Function/1(u)
  MATLAB Function/1(accel) -> Subsystem2/1(acc_cmd)
  MATLAB Function/2(decel) -> Subsystem2/2(decc_cmd)
  Subsystem2/1(T_eng_cmd) -> Gain/1
  Gain/1 -> second-order low-pass torque model/1
  Gain1/1 -> second-order low-pass brake model1/1
  Subsystem2/2(brake_cmd) -> Gain1/1
